simulink model "automata_learning"  (R2022a)
settings: Solver=FixedStepAuto  StartTime=0.0  StopTime=10.0  FixedStep=0.01  RelTol=1e-3
settings Model: Creator=diego  LastModifiedBy=diego

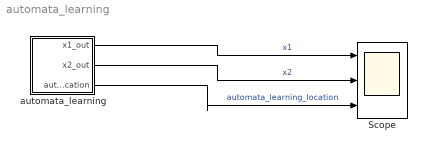
== system automata_learning ==
  Scope : Scope  NumInputPorts=3
  automata_learning : Stateflow chart  TreatAsAtomicUnit=on
  wires:
  automata_learning/1(x1_out) -> Scope/1  "x1"
  automata_learning/2(x2_out) -> Scope/2  "x2"
  automata_learning/3(automata_learning_location) -> Scope/3  "automata_learning_location"

== stateflow chart automata_learning/automata_learning ==
  settings: updateMethod=CONTINUOUS
  state loc1
    du:
    x1_dot = 88876360533815.0 * x1 / 147573952589676410000.0 - 4503601527180519.0 * x2 / 4503599627370496.0 + 189249378953091.0 * x1 * x2 / 295147905179352830000.0 + 713564437530169.0 * x1 * x2 ^ 2.0 / 4722366482869645000000.0 - 35399003772557.0 * x1 ^ 2.0 * x2 / 147573952589676410000.0 - 136846919796591.0 * x1 ^ 2.0 / 295147905179352830000.0 + 52805250175765.0 * x1 ^ 3.0 / 2361183241434822600000.0 - 769316023567919.0 * x2 ^ 2.0 / 4722366482869645000000.0 - 72353872369081.0 * x2 ^ 3.0 / 37778931862957160000000.0 - 0.00000023902594432375955;
    x2_dot = 19149947065981.0 * x2 / 295147905179352830000.0 - 3085087973773.0 * x1 / 36893488147419103000.0 - 9798790903019.0 * x1 * x2 / 36893488147419103000.0 - 48141044947291.0 * x1 * x2 ^ 2.0 / 590295810358705650000.0 + 3033604337673.0 * x1 ^ 2.0 * x2 / 590295810358705650000.0 + 140737568421071.0 * x1 ^ 2.0 / 140737488355328.0 - 313239572231841.0 * x1 ^ 3.0 / 1180591620717411300000.0 + 31003350270971.0 * x2 ^ 2.0 / 295147905179352830000.0 + 14592327137889.0 * x2 ^ 3.0 / 2361183241434822600000.0 - 0.0000002644327642465978;
    x1_out=x1;
    x2_out=x2;
    automata_learning_location =1;
  state loc2
    du:
    x1_dot = 8391434697.0 * x1 * x2 / 1125899906842624.0 - 562946737759127.0 * x2 / 562949953421312.0 - 1693660721.0 * x1 / 35184372088832.0 - 2760323619.0 * x1 * x2 ^ 2.0 / 4503599627370496.0 + 5475993885.0 * x1 ^ 2.0 * x2 / 2251799813685248.0 - 2810916777.0 * x1 ^ 2.0 / 70368744177664.0 - 186810931455.0 * x1 ^ 3.0 / 18014398509481984.0 - 797591781.0 * x2 ^ 2.0 / 562949953421312.0 - 1385999901.0 * x2 ^ 3.0 / 36028797018963968.0 - 0.000015448780583682264;
    x2_dot = 31615931071.0 * x1 * x2 ^ 2.0 / 9007199254740992.0 - 5762704953.0 * x2 / 2251799813685248.0 - 14215404889.0 * x1 * x2 / 2251799813685248.0 - 161264613819.0 * x1 / 562949953421312.0 - 34686903389.0 * x1 ^ 2.0 * x2 / 9007199254740992.0 - 1544930648505.0 * x1 ^ 2.0 / 9007199254740992.0 + 2251722159031675.0 * x1 ^ 3.0 / 2251799813685248.0 + 12593830779.0 * x2 ^ 2.0 / 2251799813685248.0 - 1249229495.0 * x2 ^ 3.0 / 18014398509481984.0 - 0.0001607949217650173;
    x1_out=x1;
    x2_out=x2;
    automata_learning_location =2;
  loc1 -> loc2 : [0.3288 * x1 - 0.333 * x2 + 1.0 < 0.0]
  (default) -> loc1 : {x1 = 1.0;
      | x2 = -1.0;}
  loc2 -> loc1 : [0.499 * x2 - 0.0006802 * x1 + 1.0 < 0.0]
  data: x1_out output; x1 local; x2_out output; x2 local; automata_learning_location output
  data x1 settings: updateMethod=SF_CONTINUOUS_TIME_DATA
  data x2 settings: updateMethod=SF_CONTINUOUS_TIME_DATA
